simulink model "PruebaN20"  (R2024b)
settings: Solver=FixedStepAuto  StartTime=0.0  StopTime=inf  RelTol=1e-3  EnableMultiTasking=on
libraries: arduinolib x8
settings Model: ExtModeTrigDuration=2  Creator=johan  LastModifiedBy=johan
settings SolverCC: AutoInsertRateTranBlk=on
settings OptimizationCC: EnhancedBackFolding=on  PassReuseOutputArgsAs=Individual arguments  ZeroExternalMemoryAtStartup=off  ZeroInternalMemoryAtStartup=off  MaxStackSize=64  OptimizeBlockOrder=speed  DifferentSizesBufferReuse=on  OptimizationCustomize=off  EfficientTunableParamExpr=on
settings DebuggingCC: ParameterTunabilityLossMsg=error
settings HardwareCC: ProdBitPerPointer=32  ProdBitPerSizeT=32  ProdBitPerPtrDiffT=32  ProdLargestAtomicInteger=Long  ProdLargestAtomicFloat=Double  ProdWordSize=32  ProdHWDeviceType=ARM Compatible->ARM Cortex
settings SFSimCC: MATLABDynamicMemAlloc=off
settings RTWCC: Description=Embedded Coder  SystemTargetFile=ert.tlc  HardwareBoard=ESP32-WROOM(Arduino Compatible)  TLCOptions="-aInlineSetEventsForThisBaseRateFcn=TLC_FALSE -aSuppressMultiTaskScheduler=TLC_FALSE  -aRateBasedStepFcn=0"  TemplateMakefile=ert_default_tmf  Toolchain=ESP32  BuildConfiguration=Faster Runs
settings CodeAppCC: ForceParamTrailComments=on  IgnoreCustomStorageClasses=off  OperatorAnnotations=on  SimulinkDataObjDesc=on  SFDataObjDesc=on  InsertBlockDesc=on
settings ERTTargetCC: SupportContinuousTime=on  SupportVariableSizeSignals=on  ExtModeTransport=3  ExtModeStaticAlloc=on  ExtModeAutomaticAllocSize=off  ExtModeStaticAllocSize=65536  ExtModeMexFile=ext_xcp  ExtModeIntrfLevel=Level2 - Open  InlinedParameterPlacement=Hierarchical

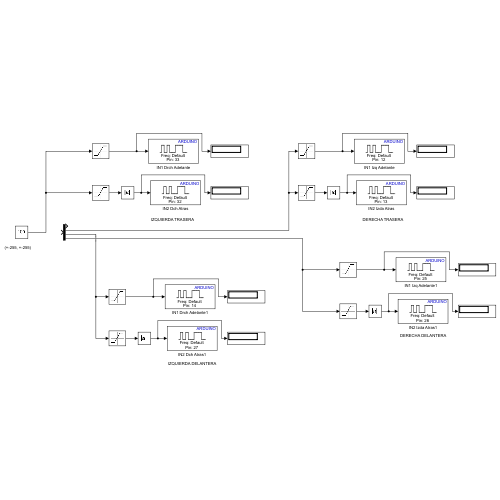
[thumbnail: Simulink's stored preview of the top-level diagram]
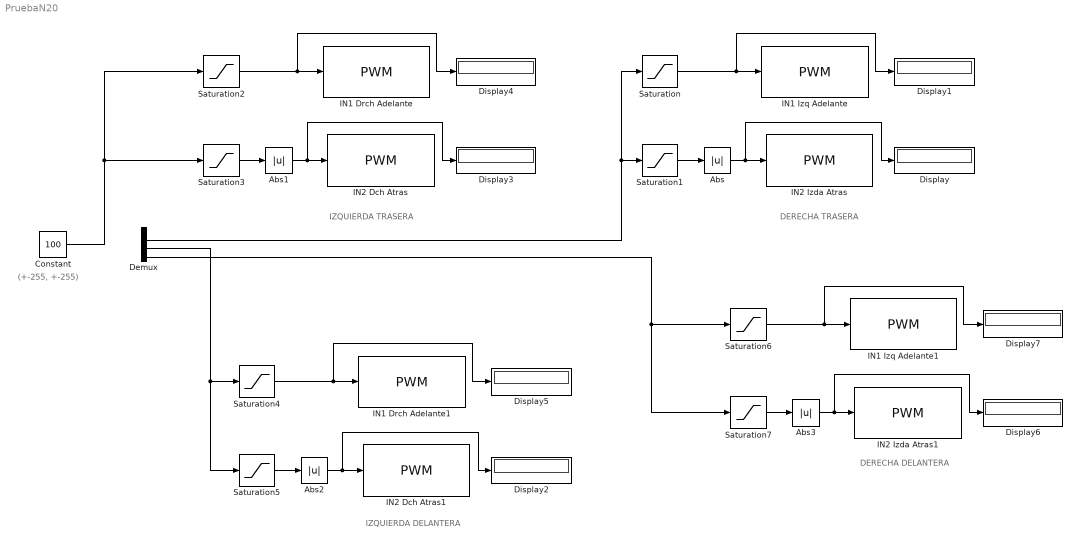
== system PruebaN20 ==
  note: (+-255, +-255)
  note: DERECHA TRASERA
  note: IZQUIERDA TRASERA
  note: IZQUIERDA DELANTERA
  note: DERECHA DELANTERA
  Abs{,1..3} (4 alike) : Abs  SaturateOnIntegerOverflow=off
  Constant : Constant  Value=100
  Demux : Demux
  Display{,1..7} (8 alike) : Display
  IN1 Drch Adelante : arduinolib/PWM  pinNumber=33  frequencyType=Default  desiredFrequency=490.2  achievableFrequency=490.2
      settings: SourceProductName=Common
  IN1 Drch Adelante1 : arduinolib/PWM  pinNumber=14  frequencyType=Default  desiredFrequency=490.2  achievableFrequency=490.2
      settings: SourceProductName=Common
  IN1 Izq Adelante : arduinolib/PWM  pinNumber=12  frequencyType=Default  desiredFrequency=490.2  achievableFrequency=490.2
      settings: SourceProductName=Common
  IN1 Izq Adelante1 : arduinolib/PWM  pinNumber=25  frequencyType=Default  desiredFrequency=490.2  achievableFrequency=490.2
      settings: SourceProductName=Common
  IN2 Dch Atras : arduinolib/PWM  pinNumber=32  frequencyType=Default  desiredFrequency=490.2  achievableFrequency=490.2
      settings: SourceProductName=Common
  IN2 Dch Atras1 : arduinolib/PWM  pinNumber=27  frequencyType=Default  desiredFrequency=490.2  achievableFrequency=490.2
      settings: SourceProductName=Common
  IN2 Izda Atras : arduinolib/PWM  pinNumber=13  frequencyType=Default  desiredFrequency=490.2  achievableFrequency=490.2
      settings: SourceProductName=Common
  IN2 Izda Atras1 : arduinolib/PWM  pinNumber=26  frequencyType=Default  desiredFrequency=490.2  achievableFrequency=490.2
      settings: SourceProductName=Common
  Saturation{,2,4,6} (4 alike) : Saturate  UpperLimit=255  LowerLimit=1
  Saturation{1,3,5,7} (4 alike) : Saturate  UpperLimit=0  LowerLimit=-255
  wires:
  Abs1/1 -> IN2 Dch Atras/1, Display3/1
  Saturation1/1 -> Abs/1
  Abs/1 -> Display/1, IN2 Izda Atras/1
  Saturation2/1 -> Display4/1, IN1 Drch Adelante/1
  Saturation3/1 -> Abs1/1
  Saturation/1 -> IN1 Izq Adelante/1, Display1/1
  Demux/3 -> Saturation5/1, Saturation4/1
  Abs2/1 -> IN2 Dch Atras1/1, Display2/1
  Saturation4/1 -> Display5/1, IN1 Drch Adelante1/1
  Saturation5/1 -> Abs2/1
  Demux/2 -> Saturation1/1, Saturation/1
  Abs3/1 -> Display6/1, IN2 Izda Atras1/1
  Saturation6/1 -> IN1 Izq Adelante1/1, Display7/1
  Saturation7/1 -> Abs3/1
  Demux/4 -> Saturation6/1, Saturation7/1
  Constant/1 -> Saturation3/1, Saturation2/1
